simulink model "TST_RngMod_TrqCalc"  (R2016b)
settings: Solver=FixedStepDiscrete  StartTime=0.0  StopTime=simTime  FixedStep=sampleTime  RelTol=1e-3
values from neighbouring files (symbols this model uses):
  testCase = 1    [initTST_RngMod_TrqCalc_001.m]
libraries: simulink x2
settings Model: Creator=wolf072601  LastModifiedBy=wolf072601
settings DebuggingCC: SignalRangeChecking=error

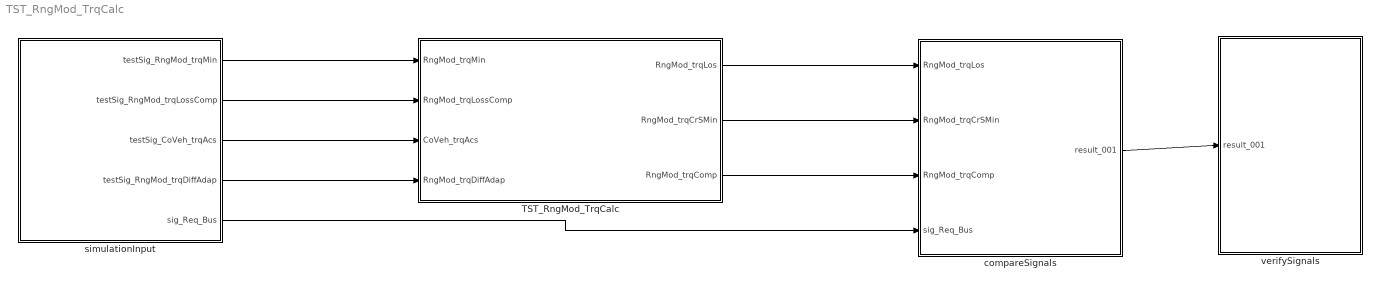
== system TST_RngMod_TrqCalc ==
  TST_RngMod_TrqCalc : Subsystem
  compareSignals : Subsystem
  simulationInput : Subsystem
  verifySignals : Subsystem
  wires:
  simulationInput/1(testSig_RngMod_trqMin) -> TST_RngMod_TrqCalc/1(RngMod_trqMin)
  simulationInput/2(testSig_RngMod_trqLossComp) -> TST_RngMod_TrqCalc/2(RngMod_trqLossComp)
  simulationInput/3(testSig_CoVeh_trqAcs) -> TST_RngMod_TrqCalc/3(CoVeh_trqAcs)
  simulationInput/4(testSig_RngMod_trqDiffAdap) -> TST_RngMod_TrqCalc/4(RngMod_trqDiffAdap)
  TST_RngMod_TrqCalc/1(RngMod_trqLos) -> compareSignals/1(RngMod_trqLos)
  TST_RngMod_TrqCalc/2(RngMod_trqCrSMin) -> compareSignals/2(RngMod_trqCrSMin)
  TST_RngMod_TrqCalc/3(RngMod_trqComp) -> compareSignals/3(RngMod_trqComp)
  simulationInput/5(sig_Req_Bus) -> compareSignals/4(sig_Req_Bus)
  compareSignals/1(result_001) -> verifySignals/1(result_001)

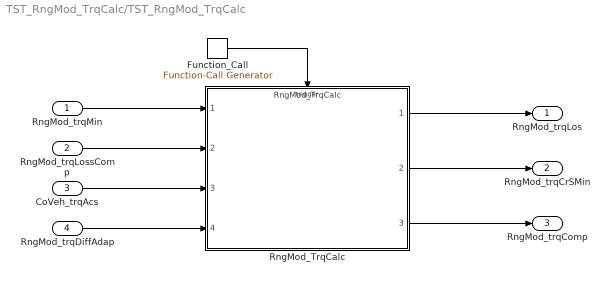
== system TST_RngMod_TrqCalc/TST_RngMod_TrqCalc ==
  RngMod_trqMin : Inport
  RngMod_trqLossComp : Inport  Port=2
  CoVeh_trqAcs : Inport  Port=3
  RngMod_trqDiffAdap : Inport  Port=4
  Function_Call : simulink/Ports & Subsystems/Function-Call Generator  sample_time=sampleTime  numberOfIterations=1
  RngMod_TrqCalc : ModelReference  ModelNameDialog=RngMod_TrqCalc  ModelReferenceVersion=1.3  TriggerPortName=function  TriggerPortTriggerType=function-call  TriggerPortStatesWhenEnabling=held
  RngMod_trqLos : Outport
  RngMod_trqCrSMin : Outport  Port=2
  RngMod_trqComp : Outport  Port=3
  wires:
  Function_Call/1 -> RngMod_TrqCalc/Trigger
  RngMod_trqMin/1 -> RngMod_TrqCalc/1
  RngMod_trqLossComp/1 -> RngMod_TrqCalc/2
  CoVeh_trqAcs/1 -> RngMod_TrqCalc/3
  RngMod_trqDiffAdap/1 -> RngMod_TrqCalc/4
  RngMod_TrqCalc/1 -> RngMod_trqLos/1
  RngMod_TrqCalc/2 -> RngMod_trqCrSMin/1
  RngMod_TrqCalc/3 -> RngMod_trqComp/1

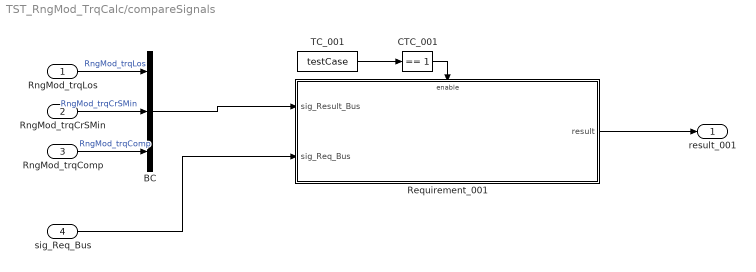
== system TST_RngMod_TrqCalc/compareSignals ==
  RngMod_trqLos : Inport
  RngMod_trqCrSMin : Inport  Port=2
  RngMod_trqComp : Inport  Port=3
  sig_Req_Bus : Inport  Port=4
  BC : BusCreator  Inputs=3
  CTC_001 : simulink/Logic and Bit Operations/Compare To Constant  relop===  const=1  OutDataTypeStr=boolean
  Requirement_001 : Subsystem
  TC_001 : Constant  Value=testCase
  result_001 : Outport
  wires:
  RngMod_trqLos/1 -> BC/1  "RngMod_trqLos"
  RngMod_trqCrSMin/1 -> BC/2  "RngMod_trqCrSMin"
  RngMod_trqComp/1 -> BC/3  "RngMod_trqComp"
  TC_001/1 -> CTC_001/1
  CTC_001/1 -> Requirement_001/Enable
  sig_Req_Bus/1 -> Requirement_001/2(sig_Req_Bus)
  BC/1 -> Requirement_001/1(sig_Result_Bus)
  Requirement_001/1(result) -> result_001/1

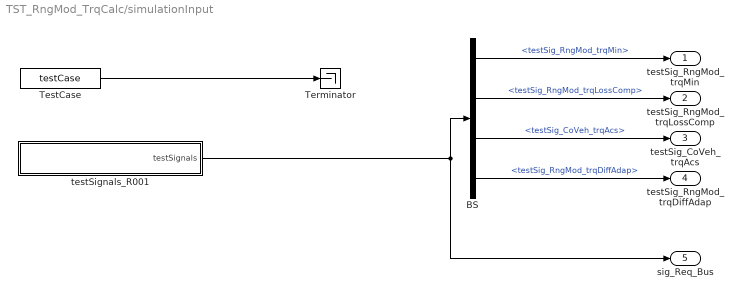
== system TST_RngMod_TrqCalc/simulationInput ==
  BS : BusSelector  OutputSignals=testSig_RngMod_trqMin,testSig_RngMod_trqLossComp,testSig_CoVeh_trqAcs,testSig_RngMod_trqDiffAdap
  Terminator : Terminator
  TestCase : Constant  Value=testCase
  testSignals_R001 : Subsystem
  testSig_RngMod_trqMin : Outport
  testSig_RngMod_trqLossComp : Outport  Port=2
  testSig_CoVeh_trqAcs : Outport  Port=3
  testSig_RngMod_trqDiffAdap : Outport  Port=4
  sig_Req_Bus : Outport  Port=5
  wires:
  BS/1 -> testSig_RngMod_trqMin/1  "<testSig_RngMod_trqMin>"
  BS/2 -> testSig_RngMod_trqLossComp/1  "<testSig_RngMod_trqLossComp>"
  BS/3 -> testSig_CoVeh_trqAcs/1  "<testSig_CoVeh_trqAcs>"
  BS/4 -> testSig_RngMod_trqDiffAdap/1  "<testSig_RngMod_trqDiffAdap>"
  testSignals_R001/1(testSignals) -> BS/1, sig_Req_Bus/1
  TestCase/1 -> Terminator/1

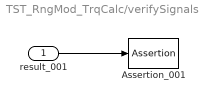
== system TST_RngMod_TrqCalc/verifySignals ==
  result_001 : Inport
  Assertion_001 : Assertion  Enabled=off
  wires:
  result_001/1 -> Assertion_001/1

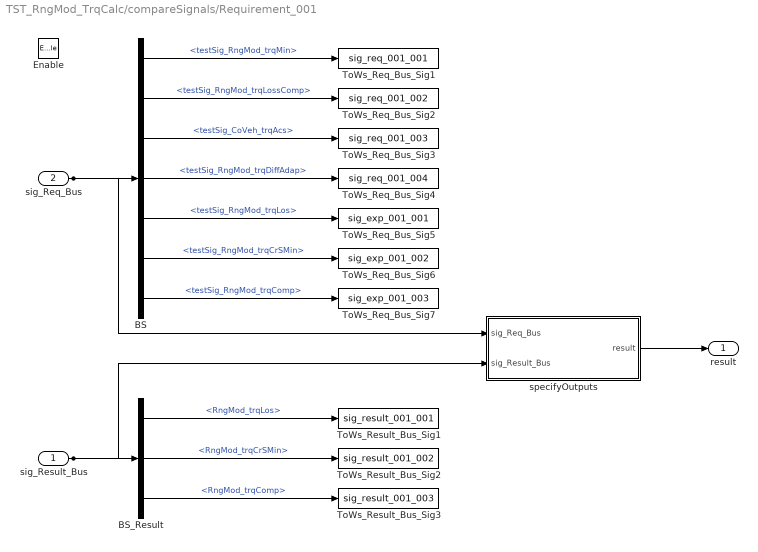
== system TST_RngMod_TrqCalc/compareSignals/Requirement_001 ==
  sig_Result_Bus : Inport
  sig_Req_Bus : Inport  Port=2
  Enable : EnablePort
  BS : BusSelector  OutputSignals=testSig_RngMod_trqMin,testSig_RngMod_trqLossComp,testSig_CoVeh_trqAcs,testSig_RngMod_trqDiffAdap,testSig_RngMod_trqLos,testSig_RngMod_trqCrSMin,testSig_RngMod_trqComp
  BS_Result : BusSelector  OutputSignals=RngMod_trqLos,RngMod_trqCrSMin,RngMod_trqComp
  ToWs_Req_Bus_Sig1 : ToWorkspace  VariableName=sig_req_001_001  SaveFormat=Structure With Time
  ToWs_Req_Bus_Sig2 : ToWorkspace  VariableName=sig_req_001_002  SaveFormat=Structure With Time
  ToWs_Req_Bus_Sig3 : ToWorkspace  VariableName=sig_req_001_003  SaveFormat=Structure With Time
  ToWs_Req_Bus_Sig4 : ToWorkspace  VariableName=sig_req_001_004  SaveFormat=Structure With Time
  ToWs_Req_Bus_Sig5 : ToWorkspace  VariableName=sig_exp_001_001  SaveFormat=Structure With Time
  ToWs_Req_Bus_Sig6 : ToWorkspace  VariableName=sig_exp_001_002  SaveFormat=Structure With Time
  ToWs_Req_Bus_Sig7 : ToWorkspace  VariableName=sig_exp_001_003  SaveFormat=Structure With Time
  ToWs_Result_Bus_Sig1 : ToWorkspace  VariableName=sig_result_001_001  SaveFormat=Structure With Time
  ToWs_Result_Bus_Sig2 : ToWorkspace  VariableName=sig_result_001_002  SaveFormat=Structure With Time
  ToWs_Result_Bus_Sig3 : ToWorkspace  VariableName=sig_result_001_003  SaveFormat=Structure With Time
  specifyOutputs : Subsystem
  result : Outport
  wires:
  sig_Req_Bus/1 -> BS/1, specifyOutputs/1(sig_Req_Bus)
  BS/1 -> ToWs_Req_Bus_Sig1/1  "<testSig_RngMod_trqMin>"
  BS/2 -> ToWs_Req_Bus_Sig2/1  "<testSig_RngMod_trqLossComp>"
  BS/3 -> ToWs_Req_Bus_Sig3/1  "<testSig_CoVeh_trqAcs>"
  BS/4 -> ToWs_Req_Bus_Sig4/1  "<testSig_RngMod_trqDiffAdap>"
  BS/5 -> ToWs_Req_Bus_Sig5/1  "<testSig_RngMod_trqLos>"
  BS/6 -> ToWs_Req_Bus_Sig6/1  "<testSig_RngMod_trqCrSMin>"
  BS/7 -> ToWs_Req_Bus_Sig7/1  "<testSig_RngMod_trqComp>"
  sig_Result_Bus/1 -> BS_Result/1, specifyOutputs/2(sig_Result_Bus)
  BS_Result/1 -> ToWs_Result_Bus_Sig1/1  "<RngMod_trqLos>"
  BS_Result/2 -> ToWs_Result_Bus_Sig2/1  "<RngMod_trqCrSMin>"
  BS_Result/3 -> ToWs_Result_Bus_Sig3/1  "<RngMod_trqComp>"
  specifyOutputs/1(result) -> result/1

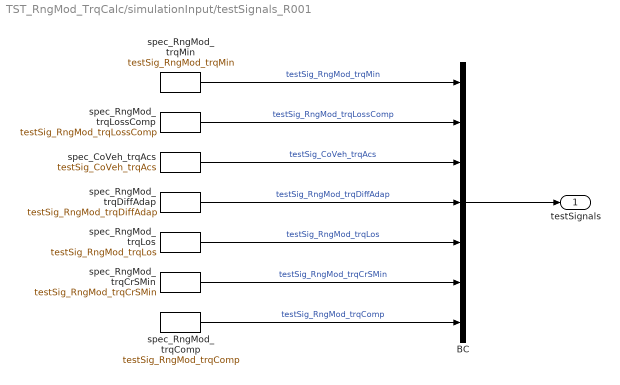
== system TST_RngMod_TrqCalc/simulationInput/testSignals_R001 ==
  BC : BusCreator  Inputs=7
  spec_CoVeh_trqAcs : FromWorkspace  VariableName=testSig_CoVeh_trqAcs  Interpolate=off  OutputAfterFinalValue=Holding final value
  spec_RngMod_trqComp : FromWorkspace  VariableName=testSig_RngMod_trqComp  Interpolate=off  OutputAfterFinalValue=Holding final value
  spec_RngMod_trqCrSMin : FromWorkspace  VariableName=testSig_RngMod_trqCrSMin  Interpolate=off  OutputAfterFinalValue=Holding final value
  spec_RngMod_trqDiffAdap : FromWorkspace  VariableName=testSig_RngMod_trqDiffAdap  Interpolate=off  OutputAfterFinalValue=Holding final value
  spec_RngMod_trqLos : FromWorkspace  VariableName=testSig_RngMod_trqLos  Interpolate=off  OutputAfterFinalValue=Holding final value
  spec_RngMod_trqLossComp : FromWorkspace  VariableName=testSig_RngMod_trqLossComp  Interpolate=off  OutputAfterFinalValue=Holding final value
  spec_RngMod_trqMin : FromWorkspace  VariableName=testSig_RngMod_trqMin  Interpolate=off  OutputAfterFinalValue=Holding final value
  testSignals : Outport
  wires:
  BC/1 -> testSignals/1
  spec_RngMod_trqMin/1 -> BC/1  "testSig_RngMod_trqMin"
  spec_RngMod_trqLossComp/1 -> BC/2  "testSig_RngMod_trqLossComp"
  spec_CoVeh_trqAcs/1 -> BC/3  "testSig_CoVeh_trqAcs"
  spec_RngMod_trqDiffAdap/1 -> BC/4  "testSig_RngMod_trqDiffAdap"
  spec_RngMod_trqLos/1 -> BC/5  "testSig_RngMod_trqLos"
  spec_RngMod_trqCrSMin/1 -> BC/6  "testSig_RngMod_trqCrSMin"
  spec_RngMod_trqComp/1 -> BC/7  "testSig_RngMod_trqComp"

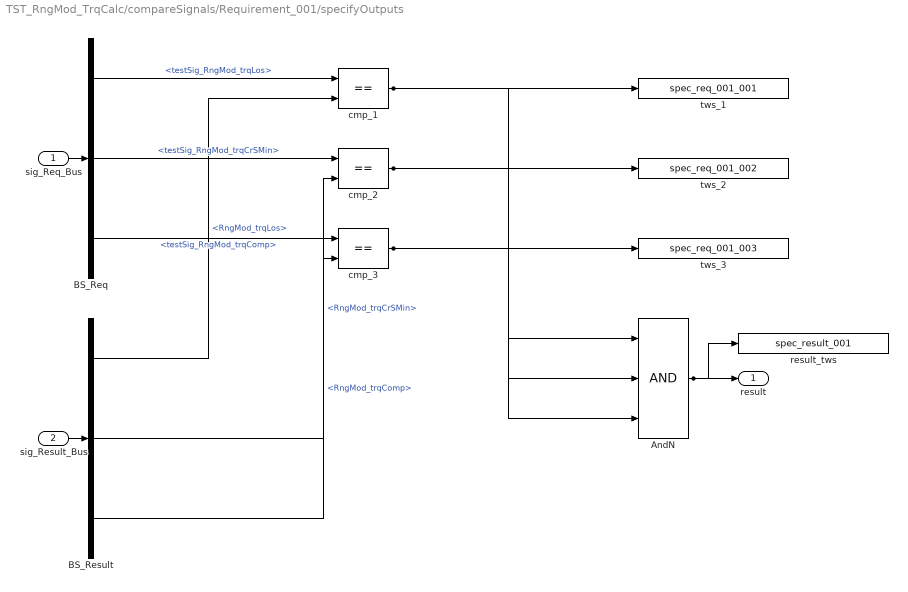
== system TST_RngMod_TrqCalc/compareSignals/Requirement_001/specifyOutputs ==
  sig_Req_Bus : Inport
  sig_Result_Bus : Inport  Port=2
  AndN : Logic  Inputs=3
  BS_Req : BusSelector  OutputSignals=testSig_RngMod_trqLos,testSig_RngMod_trqCrSMin,testSig_RngMod_trqComp
  BS_Result : BusSelector  OutputSignals=RngMod_trqLos,RngMod_trqCrSMin,RngMod_trqComp
  cmp_1 : RelationalOperator  Operator===  RndMeth=Nearest  InputSameDT=on
  cmp_2 : RelationalOperator  Operator===  RndMeth=Nearest  InputSameDT=on
  cmp_3 : RelationalOperator  Operator===  RndMeth=Nearest  InputSameDT=on
  result_tws : ToWorkspace  VariableName=spec_result_001
  tws_1 : ToWorkspace  VariableName=spec_req_001_001
  tws_2 : ToWorkspace  VariableName=spec_req_001_002
  tws_3 : ToWorkspace  VariableName=spec_req_001_003
  result : Outport
  wires:
  sig_Req_Bus/1 -> BS_Req/1
  sig_Result_Bus/1 -> BS_Result/1
  AndN/1 -> result/1, result_tws/1
  BS_Req/1 -> cmp_1/1  "<testSig_RngMod_trqLos>"
  BS_Result/1 -> cmp_1/2  "<RngMod_trqLos>"
  cmp_1/1 -> tws_1/1, AndN/1
  BS_Req/2 -> cmp_2/1  "<testSig_RngMod_trqCrSMin>"
  BS_Result/2 -> cmp_2/2  "<RngMod_trqCrSMin>"
  cmp_2/1 -> tws_2/1, AndN/2
  BS_Req/3 -> cmp_3/1  "<testSig_RngMod_trqComp>"
  BS_Result/3 -> cmp_3/2  "<RngMod_trqComp>"
  cmp_3/1 -> tws_3/1, AndN/3
